simulink subsystem "set_point_DISCRETO"  (R2023b)
settings: Solver=VariableStepAuto  StartTime=0.0  StopTime=10.0  RelTol=1e-3
values from neighbouring files (symbols this model uses):
  r = 120    [constantes.m]
settings Model: Creator=Nahuel  LastModifiedBy=rodri

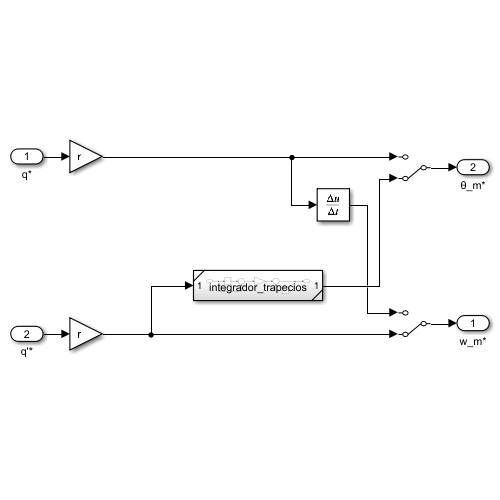
[thumbnail: Simulink's stored preview of the top-level diagram]
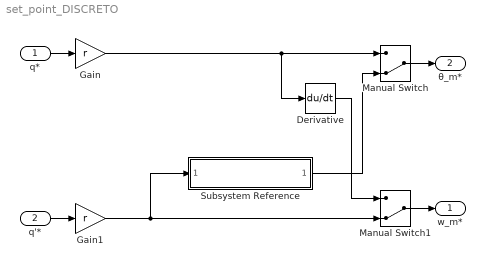
== system set_point_DISCRETO ==
  q* : Inport
  q'* : Inport  Port=2
  Derivative : Derivative
  Gain : Gain  Gain=r
  Gain1 : Gain  Gain=r
  Manual Switch : ManualSwitch  CurrentSetting=0
  Manual Switch1 : ManualSwitch  CurrentSetting=0
  Subsystem Reference : Subsystem  ReferencedSubsystem=integrador_trapecios
  w_m* : Outport
  θ_m* : Outport  Port=2
  wires:
  q*/1 -> Gain/1
  Gain/1 -> Manual Switch/1, Derivative/1
  q'*/1 -> Gain1/1
  Gain1/1 -> Subsystem Reference/1, Manual Switch1/2
  Subsystem Reference/1 -> Manual Switch/2
  Manual Switch/1 -> θ_m*/1
  Derivative/1 -> Manual Switch1/1
  Manual Switch1/1 -> w_m*/1
